simulink model "pendulum_balance_path_follow"  (R2022a)
settings: Solver=VariableStepAuto  StartTime=0.0  StopTime=100  RelTol=1e-3
libraries: simulink x1
settings Model: Creator=anthony  LastModifiedBy=anthony

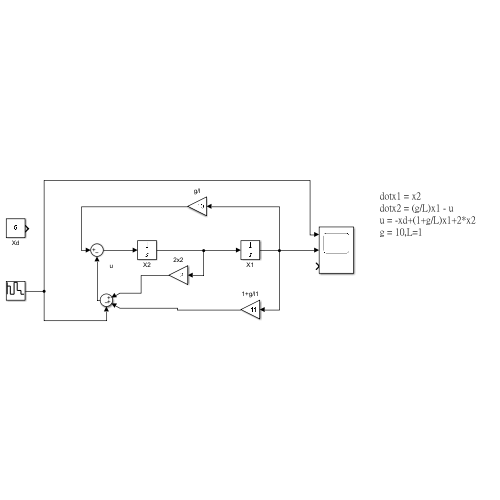
[thumbnail: Simulink's stored preview of the top-level diagram]
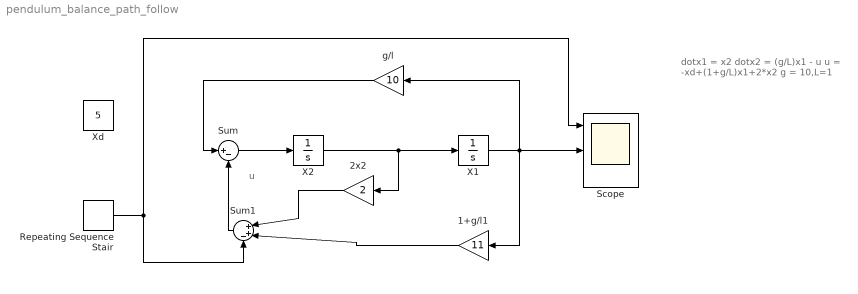
== system pendulum_balance_path_follow ==
  note: u
  note: dotx1 = x2
      | dotx2 = (g/L)x1 - u
      | u = -xd+(1+g/L)x1+2*x2
      | g = 10,L=1
  1+g/l1 : Gain  Gain=11
  2x2 : Gain  Gain=2
  Repeating Sequence Stair : simulink/Sources/Repeating Sequence Stair  OutValues=[3 1 4 2 1].'  tsamp=20  OutMin=[]  OutMax=[]  OutDataTypeStr=double  OutputDataTypeScalingMode=double  OutDataType=fixdt(0,8)  ConRadixGroup=Best Precision: Vector-wise  OutScaling=2^-12
  Scope : Scope  NumInputPorts=3
  Sum : Sum  Inputs=|+-
  Sum1 : Sum  Inputs=|++-
  X1 : Integrator
  X2 : Integrator
  Xd : Constant  Value=5
  g/l : Gain  Gain=10
  wires:
  X2/1 -> 2x2/1, X1/1
  X1/1 -> Scope/2, 1+g/l1/1, g/l/1
  Sum/1 -> X2/1
  g/l/1 -> Sum/1
  1+g/l1/1 -> Sum1/2
  2x2/1 -> Sum1/1
  Sum1/1 -> Sum/2
  Repeating Sequence Stair/1 -> Sum1/3, Scope/1
